simulink model "pid_controller"  (R2021b)
settings: Solver=FixedStepDiscrete  StartTime=0.0  StopTime=60  FixedStep=ts  RelTol=1e-3
undefined symbols (not defined in the file or in its folder): kd, ki, kp, ll, ts, ul
settings Model: Creator=adish  LastModifiedBy=adish
settings OptimizationCC: DefaultParameterBehavior=Inlined  EnhancedBackFolding=on  BooleansAsBitfields=on  PassReuseOutputArgsAs=Individual arguments  StateBitsets=on  DataBitsets=on  ZeroExternalMemoryAtStartup=off  ZeroInternalMemoryAtStartup=off  DifferentSizesBufferReuse=on  OptimizationPriority=RAM  OptimizationCustomize=off  EfficientTunableParamExpr=on
settings DebuggingCC: ParameterTunabilityLossMsg=error
settings SFSimCC: MATLABDynamicMemAlloc=off
settings RTWCC: Description=Embedded Coder  SystemTargetFile=ert.tlc  GenCodeOnly=on  TemplateMakefile=ert_default_tmf  GenerateReport=on  IncludeHyperlinkInReport=on  LaunchReport=on  GenerateTraceInfo=on  GenerateTraceReport=on  GenerateTraceReportSl=on  GenerateTraceReportSf=on  GenerateTraceReportEml=on  GenerateWebview=on  GenerateCodeReplacementReport=on
settings CodeAppCC: ForceParamTrailComments=on  IgnoreCustomStorageClasses=off  OperatorAnnotations=on  SimulinkDataObjDesc=on  SFDataObjDesc=on  InsertBlockDesc=on
settings ERTTargetCC: TargetLangStandard=C99 (ISO)  GenerateSampleERTMain=on  InlinedParameterPlacement=NonHierarchical  ERTCustomFileTemplate=example_file_process.tlc

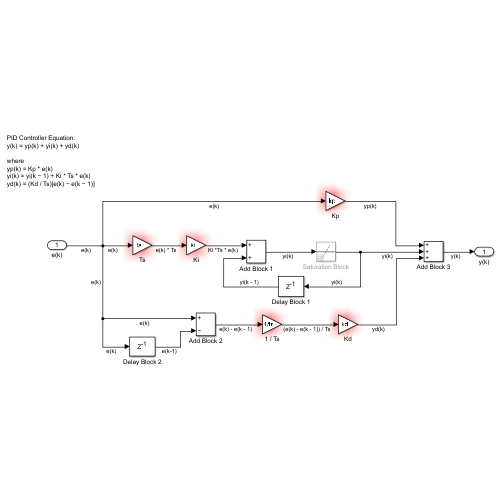
[thumbnail: Simulink's stored preview of the top-level diagram]
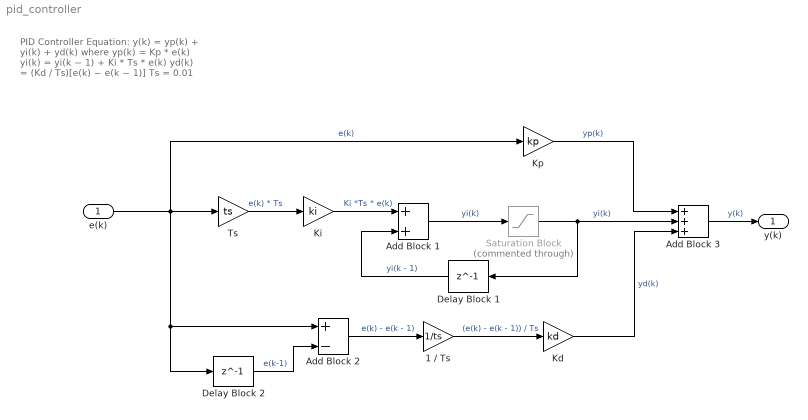
== system pid_controller ==
  note: PID Controller Equation:
      | y(k) = yp(k) + yi(k) + yd(k)
      |
      | where
      | yp(k) = Kp * e(k)
      | yi(k) = yi(k − 1) + Ki * Ts * e(k)
      | yd(k) = (Kd / Ts)[e(k) − e(k − 1)]
      | Ts = 0.01
  e(k) : Inport
  1 / Ts : Gain  Gain=1/ts
  Add Block 1 : Sum
  Add Block 2 : Sum  Inputs=+-
  Add Block 3 : Sum  Inputs=+++
  Delay Block 1 : Delay  DelayLength=1  InputProcessing=Columns as channels (frame based)  SampleTime=0.01
  Delay Block 2 : Delay  DelayLength=1  InputProcessing=Columns as channels (frame based)  SampleTime=0.01
  Kd : Gain  Gain=kd
  Ki : Gain  Gain=ki
  Kp : Gain  Gain=kp
  Saturation Block : Saturate  Commented=through  UpperLimit=ul  LowerLimit=ll
  Ts : Gain  Gain=ts
  y(k) : Outport
  wires:
  Saturation Block/1 -> Add Block 3/2, Delay Block 1/1  "yi(k)"
  Kp/1 -> Add Block 3/1  "yp(k)"
  Kd/1 -> Add Block 3/3  "yd(k)"
  Ki/1 -> Add Block 1/1  "Ki *Ts * e(k)"
  Delay Block 1/1 -> Add Block 1/2  "yi(k - 1)"
  Ts/1 -> Ki/1  "e(k) * Ts"
  Add Block 3/1 -> y(k)/1  "y(k)"
  Add Block 1/1 -> Saturation Block/1  "yi(k)"
  1 / Ts/1 -> Kd/1  "(e(k) - e(k - 1)) / Ts"
  Add Block 2/1 -> 1 / Ts/1  "e(k) - e(k - 1)"
  Delay Block 2/1 -> Add Block 2/2  "e(k-1)"
  e(k)/1 -> Kp/1, Ts/1, Add Block 2/1, Delay Block 2/1  "e(k)"
